simulink model "six_plus_six_AcmsteeringV09_main_2lflm"  (R2014a)
settings: Solver=FixedStepDiscrete  StartTime=0.0  StopTime=10.0  FixedStep=0.0005  RelTol=1e-3
InitFcn:
  | Veh_Par_wxt
undefined symbols (not defined in the file or in its folder): acc_spdctl, ag_thr, B, bra_em, bra_pre_gz2, bra_pre_gz34, bra_pre_yd, brakepre_dem_data, brakeTrq_dem_data, bratrq_max, ecucoder_acal, eff_tran, ESP_switch, G, guzhang_lf, guzhang_lm, guzhang_lr, guzhang_rf, guzhang_rm, guzhang_rr, kd1, kd2, ki1, ki2, kp1, kp2, L, myFIS, premax, Radius, RC_switch, s_opt_yi, s_opt_zhuan, s_opt_zhuan_add, s_opt_zhuan_table, spd_map_mot, spd_spdctl, speed_thr_park, TCS_switch, tras_ratio, trq_map_mot, trqmax_yd, trqmax_zx, trqmaxneg, v_gain, v_table, v_thr_park, zhidong_bianmazhi, zhidong_down, zhidong_up, zhidong_youmen, zhuanxiang_bianmazhi, zhuanxiang_down, zhuanxiang_up, zhuanxiang_youmen
libraries: simulink x980, ec5744lib x59, fuzblock x2
(part 17 of 25)

== system six_plus_six_AcmsteeringV09_main_2lflm/Data_input/BMS5_1/BMS5/BMS5_UpDownRequest_Sub ==
  In1 : Inport
  Out1 : Outport
  wires:
  In1/1 -> Out1/1

== system six_plus_six_AcmsteeringV09_main_2lflm/Data_input/BMS5_2/BMS5/BMS5_15s_InstanceDisPower_Sub ==
  In1 : Inport
  Out1 : Outport
  wires:
  In1/1 -> Out1/1

== system six_plus_six_AcmsteeringV09_main_2lflm/Data_input/BMS5_2/BMS5/BMS5_ContDischargePower_Sub ==
  In1 : Inport
  Out1 : Outport
  wires:
  In1/1 -> Out1/1

== system six_plus_six_AcmsteeringV09_main_2lflm/Data_input/BMS5_2/BMS5/BMS5_FailureLevel_Sub ==
  In1 : Inport
  Out1 : Outport
  wires:
  In1/1 -> Out1/1

== system six_plus_six_AcmsteeringV09_main_2lflm/Data_input/BMS5_2/BMS5/BMS5_FeedbackPower_Sub ==
  In1 : Inport
  Out1 : Outport
  wires:
  In1/1 -> Out1/1

== system six_plus_six_AcmsteeringV09_main_2lflm/Data_input/BMS5_2/BMS5/BMS5_UpDownRequest_Sub ==
  In1 : Inport
  Out1 : Outport
  wires:
  In1/1 -> Out1/1

== system six_plus_six_AcmsteeringV09_main_2lflm/Data_input/MCU0/MCU0/MCU0_ControlMode_Sub ==
  In1 : Inport
  Out1 : Outport
  wires:
  In1/1 -> Out1/1

== system six_plus_six_AcmsteeringV09_main_2lflm/Data_input/MCU0/MCU0/MCU0_EmergShutDown_Sub ==
  In1 : Inport
  Out1 : Outport
  wires:
  In1/1 -> Out1/1

== system six_plus_six_AcmsteeringV09_main_2lflm/Data_input/MCU0/MCU0/MCU0_GearStatus_Sub ==
  In1 : Inport
  Out1 : Outport
  wires:
  In1/1 -> Out1/1

== system six_plus_six_AcmsteeringV09_main_2lflm/Data_input/MCU0/MCU0/MCU0_HighVol_Sub ==
  In1 : Inport
  Out1 : Outport
  wires:
  In1/1 -> Out1/1

== system six_plus_six_AcmsteeringV09_main_2lflm/Data_input/MCU0/MCU0/MCU0_LiftCnt_Sub ==
  In1 : Inport
  Out1 : Outport
  wires:
  In1/1 -> Out1/1

== system six_plus_six_AcmsteeringV09_main_2lflm/Data_input/MCU0/MCU0/MCU0_ShutDowAllow_Sub ==
  In1 : Inport
  Out1 : Outport
  wires:
  In1/1 -> Out1/1

== system six_plus_six_AcmsteeringV09_main_2lflm/Data_input/MCU0/MCU0/MCU0_SpeedFdk_Sub ==
  In1 : Inport
  Out1 : Outport
  wires:
  In1/1 -> Out1/1

== system six_plus_six_AcmsteeringV09_main_2lflm/Data_input/MCU0/MCU0/MCU0_TorqueFdk_Sub ==
  In1 : Inport
  Out1 : Outport
  wires:
  In1/1 -> Out1/1

== system six_plus_six_AcmsteeringV09_main_2lflm/Data_input/MCU0/MCU0/MCU0_TorqueMax_Sub ==
  In1 : Inport
  Out1 : Outport
  wires:
  In1/1 -> Out1/1

== system six_plus_six_AcmsteeringV09_main_2lflm/Data_input/MCU0/MCU0/MCU0_WorkStatus_Sub ==
  In1 : Inport
  Out1 : Outport
  wires:
  In1/1 -> Out1/1

== system six_plus_six_AcmsteeringV09_main_2lflm/Data_input/MCU0_1/MCU0/MCU0_ControlMode_Sub ==
  In1 : Inport
  Out1 : Outport
  wires:
  In1/1 -> Out1/1

== system six_plus_six_AcmsteeringV09_main_2lflm/Data_input/MCU0_1/MCU0/MCU0_EmergShutDown_Sub ==
  In1 : Inport
  Out1 : Outport
  wires:
  In1/1 -> Out1/1

== system six_plus_six_AcmsteeringV09_main_2lflm/Data_input/MCU0_1/MCU0/MCU0_GearStatus_Sub ==
  In1 : Inport
  Out1 : Outport
  wires:
  In1/1 -> Out1/1

== system six_plus_six_AcmsteeringV09_main_2lflm/Data_input/MCU0_1/MCU0/MCU0_HighVol_Sub ==
  In1 : Inport
  Out1 : Outport
  wires:
  In1/1 -> Out1/1

== system six_plus_six_AcmsteeringV09_main_2lflm/Data_input/MCU0_1/MCU0/MCU0_LiftCnt_Sub ==
  In1 : Inport
  Out1 : Outport
  wires:
  In1/1 -> Out1/1

== system six_plus_six_AcmsteeringV09_main_2lflm/Data_input/MCU0_1/MCU0/MCU0_ShutDowAllow_Sub ==
  In1 : Inport
  Out1 : Outport
  wires:
  In1/1 -> Out1/1

== system six_plus_six_AcmsteeringV09_main_2lflm/Data_input/MCU0_1/MCU0/MCU0_SpeedFdk_Sub ==
  In1 : Inport
  Out1 : Outport
  wires:
  In1/1 -> Out1/1

== system six_plus_six_AcmsteeringV09_main_2lflm/Data_input/MCU0_1/MCU0/MCU0_TorqueFdk_Sub ==
  In1 : Inport
  Out1 : Outport
  wires:
  In1/1 -> Out1/1

== system six_plus_six_AcmsteeringV09_main_2lflm/Data_input/MCU0_1/MCU0/MCU0_TorqueMax_Sub ==
  In1 : Inport
  Out1 : Outport
  wires:
  In1/1 -> Out1/1

== system six_plus_six_AcmsteeringV09_main_2lflm/Data_input/MCU0_1/MCU0/MCU0_WorkStatus_Sub ==
  In1 : Inport
  Out1 : Outport
  wires:
  In1/1 -> Out1/1

== system six_plus_six_AcmsteeringV09_main_2lflm/Data_input/MCU0_2/MCU0/MCU0_ControlMode_Sub ==
  In1 : Inport
  Out1 : Outport
  wires:
  In1/1 -> Out1/1

== system six_plus_six_AcmsteeringV09_main_2lflm/Data_input/MCU0_2/MCU0/MCU0_EmergShutDown_Sub ==
  In1 : Inport
  Out1 : Outport
  wires:
  In1/1 -> Out1/1

== system six_plus_six_AcmsteeringV09_main_2lflm/Data_input/MCU0_2/MCU0/MCU0_GearStatus_Sub ==
  In1 : Inport
  Out1 : Outport
  wires:
  In1/1 -> Out1/1

== system six_plus_six_AcmsteeringV09_main_2lflm/Data_input/MCU0_2/MCU0/MCU0_HighVol_Sub ==
  In1 : Inport
  Out1 : Outport
  wires:
  In1/1 -> Out1/1

== system six_plus_six_AcmsteeringV09_main_2lflm/Data_input/MCU0_2/MCU0/MCU0_LiftCnt_Sub ==
  In1 : Inport
  Out1 : Outport
  wires:
  In1/1 -> Out1/1

== system six_plus_six_AcmsteeringV09_main_2lflm/Data_input/MCU0_2/MCU0/MCU0_ShutDowAllow_Sub ==
  In1 : Inport
  Out1 : Outport
  wires:
  In1/1 -> Out1/1

== system six_plus_six_AcmsteeringV09_main_2lflm/Data_input/MCU0_2/MCU0/MCU0_SpeedFdk_Sub ==
  In1 : Inport
  Out1 : Outport
  wires:
  In1/1 -> Out1/1

== system six_plus_six_AcmsteeringV09_main_2lflm/Data_input/MCU0_2/MCU0/MCU0_TorqueFdk_Sub ==
  In1 : Inport
  Out1 : Outport
  wires:
  In1/1 -> Out1/1

== system six_plus_six_AcmsteeringV09_main_2lflm/Data_input/MCU0_2/MCU0/MCU0_TorqueMax_Sub ==
  In1 : Inport
  Out1 : Outport
  wires:
  In1/1 -> Out1/1

== matlab function six_plus_six_AcmsteeringV09_main_2lflm/Data_input/10/Enabled
Subsystem/MATLAB Function ==
  data: data1 input; y output; data2 input; data3 input; data4 input
function y = fcn(data1,data2,data3,data4)
%#codegen
y1=data4*256^3+data3*256^2+data2*256+data1;
y=typecast(uint32(y1),'single');
end
% y = u;

== matlab function six_plus_six_AcmsteeringV09_main_2lflm/InputSignalProcess/MATLAB Function ==
  data: LeftJoystick_UpDown input; acc_dem output single; steer_dem output single; brake_dem output single; LeftJoystick_LeftRight input; RirhtJoystick_UpDown input
function [acc_dem,steer_dem,brake_dem] = fcn(LeftJoystick_UpDown,LeftJoystick_LeftRight,RirhtJoystick_UpDown)
%#codegen
if LeftJoystick_UpDown<=1512
    acc_dem=single((LeftJoystick_UpDown-1512)/(1094-1512)*100);
else
    acc_dem=single((LeftJoystick_UpDown-1512)/(1934-1512)*100*-1);
end

if  LeftJoystick_LeftRight <500 || LeftJoystick_LeftRight >2500
    steer_dem = single(0);
elseif LeftJoystick_LeftRight<=1503
    steer_dem=single((LeftJoystick_LeftRight-1503)/(1084-1503)*100);
else
    steer_dem=single((LeftJoystick_LeftRight-1503)/(1923-1503)*100*-1);
end

brake_dem=single((RirhtJoystick_UpDown-1094)/(1934-1094)*100);

end

== system six_plus_six_AcmsteeringV09_main_2lflm/Data_input/MCU0_2/MCU0/MCU0_WorkStatus_Sub ==
  In1 : Inport
  Out1 : Outport
  wires:
  In1/1 -> Out1/1

== system six_plus_six_AcmsteeringV09_main_2lflm/Data_input/MCU0_3/MCU0/MCU0_ControlMode_Sub ==
  In1 : Inport
  Out1 : Outport
  wires:
  In1/1 -> Out1/1

== system six_plus_six_AcmsteeringV09_main_2lflm/Data_input/MCU0_3/MCU0/MCU0_EmergShutDown_Sub ==
  In1 : Inport
  Out1 : Outport
  wires:
  In1/1 -> Out1/1

== system six_plus_six_AcmsteeringV09_main_2lflm/Data_input/MCU0_3/MCU0/MCU0_GearStatus_Sub ==
  In1 : Inport
  Out1 : Outport
  wires:
  In1/1 -> Out1/1

== system six_plus_six_AcmsteeringV09_main_2lflm/Data_input/MCU0_3/MCU0/MCU0_HighVol_Sub ==
  In1 : Inport
  Out1 : Outport
  wires:
  In1/1 -> Out1/1

== system six_plus_six_AcmsteeringV09_main_2lflm/Data_input/MCU0_3/MCU0/MCU0_LiftCnt_Sub ==
  In1 : Inport
  Out1 : Outport
  wires:
  In1/1 -> Out1/1

== system six_plus_six_AcmsteeringV09_main_2lflm/Data_input/MCU0_3/MCU0/MCU0_ShutDowAllow_Sub ==
  In1 : Inport
  Out1 : Outport
  wires:
  In1/1 -> Out1/1

== system six_plus_six_AcmsteeringV09_main_2lflm/Data_input/MCU0_3/MCU0/MCU0_SpeedFdk_Sub ==
  In1 : Inport
  Out1 : Outport
  wires:
  In1/1 -> Out1/1

== system six_plus_six_AcmsteeringV09_main_2lflm/Data_input/MCU0_3/MCU0/MCU0_TorqueFdk_Sub ==
  In1 : Inport
  Out1 : Outport
  wires:
  In1/1 -> Out1/1

== system six_plus_six_AcmsteeringV09_main_2lflm/Data_input/MCU0_3/MCU0/MCU0_TorqueMax_Sub ==
  In1 : Inport
  Out1 : Outport
  wires:
  In1/1 -> Out1/1

== system six_plus_six_AcmsteeringV09_main_2lflm/Data_input/MCU0_3/MCU0/MCU0_WorkStatus_Sub ==
  In1 : Inport
  Out1 : Outport
  wires:
  In1/1 -> Out1/1

== system six_plus_six_AcmsteeringV09_main_2lflm/Data_input/MCU0_4/MCU0/MCU0_ControlMode_Sub ==
  In1 : Inport
  Out1 : Outport
  wires:
  In1/1 -> Out1/1

== system six_plus_six_AcmsteeringV09_main_2lflm/Data_input/MCU0_4/MCU0/MCU0_EmergShutDown_Sub ==
  In1 : Inport
  Out1 : Outport
  wires:
  In1/1 -> Out1/1

== system six_plus_six_AcmsteeringV09_main_2lflm/Data_input/MCU0_4/MCU0/MCU0_GearStatus_Sub ==
  In1 : Inport
  Out1 : Outport
  wires:
  In1/1 -> Out1/1

== system six_plus_six_AcmsteeringV09_main_2lflm/Data_input/MCU0_4/MCU0/MCU0_HighVol_Sub ==
  In1 : Inport
  Out1 : Outport
  wires:
  In1/1 -> Out1/1

== system six_plus_six_AcmsteeringV09_main_2lflm/Data_input/MCU0_4/MCU0/MCU0_LiftCnt_Sub ==
  In1 : Inport
  Out1 : Outport
  wires:
  In1/1 -> Out1/1

== system six_plus_six_AcmsteeringV09_main_2lflm/Data_input/MCU0_4/MCU0/MCU0_ShutDowAllow_Sub ==
  In1 : Inport
  Out1 : Outport
  wires:
  In1/1 -> Out1/1

== system six_plus_six_AcmsteeringV09_main_2lflm/Data_input/MCU0_4/MCU0/MCU0_SpeedFdk_Sub ==
  In1 : Inport
  Out1 : Outport
  wires:
  In1/1 -> Out1/1

== system six_plus_six_AcmsteeringV09_main_2lflm/Data_input/MCU0_4/MCU0/MCU0_TorqueFdk_Sub ==
  In1 : Inport
  Out1 : Outport
  wires:
  In1/1 -> Out1/1

== system six_plus_six_AcmsteeringV09_main_2lflm/Data_input/MCU0_4/MCU0/MCU0_TorqueMax_Sub ==
  In1 : Inport
  Out1 : Outport
  wires:
  In1/1 -> Out1/1

== system six_plus_six_AcmsteeringV09_main_2lflm/Data_input/MCU0_4/MCU0/MCU0_WorkStatus_Sub ==
  In1 : Inport
  Out1 : Outport
  wires:
  In1/1 -> Out1/1

== system six_plus_six_AcmsteeringV09_main_2lflm/Data_input/MCU0_5/MCU0/MCU0_ControlMode_Sub ==
  In1 : Inport
  Out1 : Outport
  wires:
  In1/1 -> Out1/1

== system six_plus_six_AcmsteeringV09_main_2lflm/Data_input/MCU0_5/MCU0/MCU0_EmergShutDown_Sub ==
  In1 : Inport
  Out1 : Outport
  wires:
  In1/1 -> Out1/1

== system six_plus_six_AcmsteeringV09_main_2lflm/Data_input/MCU0_5/MCU0/MCU0_GearStatus_Sub ==
  In1 : Inport
  Out1 : Outport
  wires:
  In1/1 -> Out1/1

== system six_plus_six_AcmsteeringV09_main_2lflm/Data_input/MCU0_5/MCU0/MCU0_HighVol_Sub ==
  In1 : Inport
  Out1 : Outport
  wires:
  In1/1 -> Out1/1

== system six_plus_six_AcmsteeringV09_main_2lflm/Data_input/MCU0_5/MCU0/MCU0_LiftCnt_Sub ==
  In1 : Inport
  Out1 : Outport
  wires:
  In1/1 -> Out1/1

== system six_plus_six_AcmsteeringV09_main_2lflm/Data_input/MCU0_5/MCU0/MCU0_ShutDowAllow_Sub ==
  In1 : Inport
  Out1 : Outport
  wires:
  In1/1 -> Out1/1

== system six_plus_six_AcmsteeringV09_main_2lflm/Data_input/MCU0_5/MCU0/MCU0_SpeedFdk_Sub ==
  In1 : Inport
  Out1 : Outport
  wires:
  In1/1 -> Out1/1

== system six_plus_six_AcmsteeringV09_main_2lflm/Data_input/MCU0_5/MCU0/MCU0_TorqueFdk_Sub ==
  In1 : Inport
  Out1 : Outport
  wires:
  In1/1 -> Out1/1

== system six_plus_six_AcmsteeringV09_main_2lflm/Data_input/MCU0_5/MCU0/MCU0_TorqueMax_Sub ==
  In1 : Inport
  Out1 : Outport
  wires:
  In1/1 -> Out1/1

== system six_plus_six_AcmsteeringV09_main_2lflm/Data_input/MCU0_5/MCU0/MCU0_WorkStatus_Sub ==
  In1 : Inport
  Out1 : Outport
  wires:
  In1/1 -> Out1/1

== system six_plus_six_AcmsteeringV09_main_2lflm/Data_input/MCU1/MCU1/MCU1_ControlTemp_Sub ==
  In1 : Inport
  Out1 : Outport
  wires:
  In1/1 -> Out1/1

== system six_plus_six_AcmsteeringV09_main_2lflm/Data_input/MCU1/MCU1/MCU1_Idc_Sub ==
  In1 : Inport
  Out1 : Outport
  wires:
  In1/1 -> Out1/1

== system six_plus_six_AcmsteeringV09_main_2lflm/Data_input/MCU1/MCU1/MCU1_MotorTemp_Sub ==
  In1 : Inport
  Out1 : Outport
  wires:
  In1/1 -> Out1/1

== system six_plus_six_AcmsteeringV09_main_2lflm/Data_input/MCU1/MCU1/MCU1_PowerFdk_Sub ==
  In1 : Inport
  Out1 : Outport
  wires:
  In1/1 -> Out1/1

== system six_plus_six_AcmsteeringV09_main_2lflm/Data_input/MCU1/MCU1/MCU1_Udc_Sub ==
  In1 : Inport
  Out1 : Outport
  wires:
  In1/1 -> Out1/1

== system six_plus_six_AcmsteeringV09_main_2lflm/Data_input/MCU1_1/MCU1/MCU1_ControlTemp_Sub ==
  In1 : Inport
  Out1 : Outport
  wires:
  In1/1 -> Out1/1

== system six_plus_six_AcmsteeringV09_main_2lflm/Data_input/MCU1_1/MCU1/MCU1_Idc_Sub ==
  In1 : Inport
  Out1 : Outport
  wires:
  In1/1 -> Out1/1

== system six_plus_six_AcmsteeringV09_main_2lflm/Data_input/MCU1_1/MCU1/MCU1_MotorTemp_Sub ==
  In1 : Inport
  Out1 : Outport
  wires:
  In1/1 -> Out1/1

== system six_plus_six_AcmsteeringV09_main_2lflm/Data_input/MCU1_1/MCU1/MCU1_PowerFdk_Sub ==
  In1 : Inport
  Out1 : Outport
  wires:
  In1/1 -> Out1/1

== system six_plus_six_AcmsteeringV09_main_2lflm/Data_input/MCU1_1/MCU1/MCU1_Udc_Sub ==
  In1 : Inport
  Out1 : Outport
  wires:
  In1/1 -> Out1/1

== system six_plus_six_AcmsteeringV09_main_2lflm/Data_input/MCU1_2/MCU1/MCU1_ControlTemp_Sub ==
  In1 : Inport
  Out1 : Outport
  wires:
  In1/1 -> Out1/1

== system six_plus_six_AcmsteeringV09_main_2lflm/Data_input/MCU1_2/MCU1/MCU1_Idc_Sub ==
  In1 : Inport
  Out1 : Outport
  wires:
  In1/1 -> Out1/1

== system six_plus_six_AcmsteeringV09_main_2lflm/Data_input/MCU1_2/MCU1/MCU1_MotorTemp_Sub ==
  In1 : Inport
  Out1 : Outport
  wires:
  In1/1 -> Out1/1

== system six_plus_six_AcmsteeringV09_main_2lflm/Data_input/MCU1_2/MCU1/MCU1_PowerFdk_Sub ==
  In1 : Inport
  Out1 : Outport
  wires:
  In1/1 -> Out1/1

== system six_plus_six_AcmsteeringV09_main_2lflm/Data_input/MCU1_2/MCU1/MCU1_Udc_Sub ==
  In1 : Inport
  Out1 : Outport
  wires:
  In1/1 -> Out1/1

== system six_plus_six_AcmsteeringV09_main_2lflm/Data_input/MCU1_3/MCU1/MCU1_ControlTemp_Sub ==
  In1 : Inport
  Out1 : Outport
  wires:
  In1/1 -> Out1/1

== system six_plus_six_AcmsteeringV09_main_2lflm/Data_input/MCU1_3/MCU1/MCU1_Idc_Sub ==
  In1 : Inport
  Out1 : Outport
  wires:
  In1/1 -> Out1/1

== system six_plus_six_AcmsteeringV09_main_2lflm/Data_input/MCU1_3/MCU1/MCU1_MotorTemp_Sub ==
  In1 : Inport
  Out1 : Outport
  wires:
  In1/1 -> Out1/1

== system six_plus_six_AcmsteeringV09_main_2lflm/Data_input/MCU1_3/MCU1/MCU1_PowerFdk_Sub ==
  In1 : Inport
  Out1 : Outport
  wires:
  In1/1 -> Out1/1

== system six_plus_six_AcmsteeringV09_main_2lflm/Data_input/MCU1_3/MCU1/MCU1_Udc_Sub ==
  In1 : Inport
  Out1 : Outport
  wires:
  In1/1 -> Out1/1

== system six_plus_six_AcmsteeringV09_main_2lflm/Data_input/MCU1_4/MCU1/MCU1_ControlTemp_Sub ==
  In1 : Inport
  Out1 : Outport
  wires:
  In1/1 -> Out1/1

== system six_plus_six_AcmsteeringV09_main_2lflm/Data_input/MCU1_4/MCU1/MCU1_Idc_Sub ==
  In1 : Inport
  Out1 : Outport
  wires:
  In1/1 -> Out1/1

== system six_plus_six_AcmsteeringV09_main_2lflm/Data_input/MCU1_4/MCU1/MCU1_MotorTemp_Sub ==
  In1 : Inport
  Out1 : Outport
  wires:
  In1/1 -> Out1/1

== system six_plus_six_AcmsteeringV09_main_2lflm/Data_input/MCU1_4/MCU1/MCU1_PowerFdk_Sub ==
  In1 : Inport
  Out1 : Outport
  wires:
  In1/1 -> Out1/1

== system six_plus_six_AcmsteeringV09_main_2lflm/Data_input/MCU1_4/MCU1/MCU1_Udc_Sub ==
  In1 : Inport
  Out1 : Outport
  wires:
  In1/1 -> Out1/1

== system six_plus_six_AcmsteeringV09_main_2lflm/Data_input/MCU1_5/MCU1/MCU1_ControlTemp_Sub ==
  In1 : Inport
  Out1 : Outport
  wires:
  In1/1 -> Out1/1

== system six_plus_six_AcmsteeringV09_main_2lflm/Data_input/MCU1_5/MCU1/MCU1_Idc_Sub ==
  In1 : Inport
  Out1 : Outport
  wires:
  In1/1 -> Out1/1

== system six_plus_six_AcmsteeringV09_main_2lflm/Data_input/MCU1_5/MCU1/MCU1_MotorTemp_Sub ==
  In1 : Inport
  Out1 : Outport
  wires:
  In1/1 -> Out1/1

== system six_plus_six_AcmsteeringV09_main_2lflm/Data_input/MCU1_5/MCU1/MCU1_PowerFdk_Sub ==
  In1 : Inport
  Out1 : Outport
  wires:
  In1/1 -> Out1/1

== system six_plus_six_AcmsteeringV09_main_2lflm/Data_input/MCU1_5/MCU1/MCU1_Udc_Sub ==
  In1 : Inport
  Out1 : Outport
  wires:
  In1/1 -> Out1/1

== system six_plus_six_AcmsteeringV09_main_2lflm/Data_input/MCU2/MCU2/MCU2_ActieDischargingFault_Sub ==
  In1 : Inport
  Out1 : Outport
  wires:
  In1/1 -> Out1/1

== system six_plus_six_AcmsteeringV09_main_2lflm/Data_input/MCU2/MCU2/MCU2_CanCommunicationFault_Sub ==
  In1 : Inport
  Out1 : Outport
  wires:
  In1/1 -> Out1/1

== system six_plus_six_AcmsteeringV09_main_2lflm/Data_input/MCU2/MCU2/MCU2_ControllerOverTemp_Sub ==
  In1 : Inport
  Out1 : Outport
  wires:
  In1/1 -> Out1/1

== system six_plus_six_AcmsteeringV09_main_2lflm/Data_input/MCU2/MCU2/MCU2_ControllerOverload_Sub ==
  In1 : Inport
  Out1 : Outport
  wires:
  In1/1 -> Out1/1

== system six_plus_six_AcmsteeringV09_main_2lflm/Data_input/MCU2/MCU2/MCU2_DownratingFault_Sub ==
  In1 : Inport
  Out1 : Outport
  wires:
  In1/1 -> Out1/1

== system six_plus_six_AcmsteeringV09_main_2lflm/Data_input/MCU2/MCU2/MCU2_FaultLevel_Sub ==
  In1 : Inport
  Out1 : Outport
  wires:
  In1/1 -> Out1/1

== system six_plus_six_AcmsteeringV09_main_2lflm/Data_input/MCU2/MCU2/MCU2_IGBTFault_Sub ==
  In1 : Inport
  Out1 : Outport
  wires:
  In1/1 -> Out1/1

== system six_plus_six_AcmsteeringV09_main_2lflm/Data_input/MCU2/MCU2/MCU2_IdcSensorFault_Sub ==
  In1 : Inport
  Out1 : Outport
  wires:
  In1/1 -> Out1/1

== system six_plus_six_AcmsteeringV09_main_2lflm/Data_input/MCU2/MCU2/MCU2_IuSensorFault_Sub ==
  In1 : Inport
  Out1 : Outport
  wires:
  In1/1 -> Out1/1

== system six_plus_six_AcmsteeringV09_main_2lflm/Data_input/MCU2/MCU2/MCU2_IvSensorFault_Sub ==
  In1 : Inport
  Out1 : Outport
  wires:
  In1/1 -> Out1/1

== system six_plus_six_AcmsteeringV09_main_2lflm/Data_input/MCU2/MCU2/MCU2_MemoryFault_Sub ==
  In1 : Inport
  Out1 : Outport
  wires:
  In1/1 -> Out1/1

== system six_plus_six_AcmsteeringV09_main_2lflm/Data_input/MCU2/MCU2/MCU2_MotorOverLoad_Sub ==
  In1 : Inport
  Out1 : Outport
  wires:
  In1/1 -> Out1/1

== system six_plus_six_AcmsteeringV09_main_2lflm/Data_input/MCU2/MCU2/MCU2_MotorOverSpeed_Sub ==
  In1 : Inport
  Out1 : Outport
  wires:
  In1/1 -> Out1/1

== system six_plus_six_AcmsteeringV09_main_2lflm/Data_input/MCU2/MCU2/MCU2_MotorOverTemp_Sub ==
  In1 : Inport
  Out1 : Outport
  wires:
  In1/1 -> Out1/1

== system six_plus_six_AcmsteeringV09_main_2lflm/Data_input/MCU2/MCU2/MCU2_MotorStallingFault_Sub ==
  In1 : Inport
  Out1 : Outport
  wires:
  In1/1 -> Out1/1

== system six_plus_six_AcmsteeringV09_main_2lflm/Data_input/MCU2/MCU2/MCU2_OverVoltage_Sub ==
  In1 : Inport
  Out1 : Outport
  wires:
  In1/1 -> Out1/1

== system six_plus_six_AcmsteeringV09_main_2lflm/Data_input/MCU2/MCU2/MCU2_RotaryInverterFault_Sub ==
  In1 : Inport
  Out1 : Outport
  wires:
  In1/1 -> Out1/1

== system six_plus_six_AcmsteeringV09_main_2lflm/Data_input/MCU2/MCU2/MCU2_TempSensorFault_Sub ==
  In1 : Inport
  Out1 : Outport
  wires:
  In1/1 -> Out1/1

== system six_plus_six_AcmsteeringV09_main_2lflm/Data_input/MCU2/MCU2/MCU2_UdcDetectionFault_Sub ==
  In1 : Inport
  Out1 : Outport
  wires:
  In1/1 -> Out1/1

== system six_plus_six_AcmsteeringV09_main_2lflm/Data_input/MCU2/MCU2/MCU2_UnderVoltage_Sub ==
  In1 : Inport
  Out1 : Outport
  wires:
  In1/1 -> Out1/1

== system six_plus_six_AcmsteeringV09_main_2lflm/Data_input/MCU2_1/MCU2/MCU2_ActieDischargingFault_Sub ==
  In1 : Inport
  Out1 : Outport
  wires:
  In1/1 -> Out1/1

== system six_plus_six_AcmsteeringV09_main_2lflm/Data_input/MCU2_1/MCU2/MCU2_CanCommunicationFault_Sub ==
  In1 : Inport
  Out1 : Outport
  wires:
  In1/1 -> Out1/1

== system six_plus_six_AcmsteeringV09_main_2lflm/Data_input/MCU2_1/MCU2/MCU2_ControllerOverTemp_Sub ==
  In1 : Inport
  Out1 : Outport
  wires:
  In1/1 -> Out1/1

== system six_plus_six_AcmsteeringV09_main_2lflm/Data_input/MCU2_1/MCU2/MCU2_ControllerOverload_Sub ==
  In1 : Inport
  Out1 : Outport
  wires:
  In1/1 -> Out1/1

== system six_plus_six_AcmsteeringV09_main_2lflm/Data_input/MCU2_1/MCU2/MCU2_DownratingFault_Sub ==
  In1 : Inport
  Out1 : Outport
  wires:
  In1/1 -> Out1/1

== system six_plus_six_AcmsteeringV09_main_2lflm/Data_input/MCU2_1/MCU2/MCU2_FaultLevel_Sub ==
  In1 : Inport
  Out1 : Outport
  wires:
  In1/1 -> Out1/1

== system six_plus_six_AcmsteeringV09_main_2lflm/Data_input/MCU2_1/MCU2/MCU2_IGBTFault_Sub ==
  In1 : Inport
  Out1 : Outport
  wires:
  In1/1 -> Out1/1

== system six_plus_six_AcmsteeringV09_main_2lflm/Data_input/MCU2_1/MCU2/MCU2_IdcSensorFault_Sub ==
  In1 : Inport
  Out1 : Outport
  wires:
  In1/1 -> Out1/1

== system six_plus_six_AcmsteeringV09_main_2lflm/Data_input/MCU2_1/MCU2/MCU2_IuSensorFault_Sub ==
  In1 : Inport
  Out1 : Outport
  wires:
  In1/1 -> Out1/1

== system six_plus_six_AcmsteeringV09_main_2lflm/Data_input/MCU2_1/MCU2/MCU2_IvSensorFault_Sub ==
  In1 : Inport
  Out1 : Outport
  wires:
  In1/1 -> Out1/1

== system six_plus_six_AcmsteeringV09_main_2lflm/Data_input/MCU2_1/MCU2/MCU2_MemoryFault_Sub ==
  In1 : Inport
  Out1 : Outport
  wires:
  In1/1 -> Out1/1

== system six_plus_six_AcmsteeringV09_main_2lflm/Data_input/MCU2_1/MCU2/MCU2_MotorOverLoad_Sub ==
  In1 : Inport
  Out1 : Outport
  wires:
  In1/1 -> Out1/1

== system six_plus_six_AcmsteeringV09_main_2lflm/Data_input/MCU2_1/MCU2/MCU2_MotorOverSpeed_Sub ==
  In1 : Inport
  Out1 : Outport
  wires:
  In1/1 -> Out1/1

== system six_plus_six_AcmsteeringV09_main_2lflm/Data_input/MCU2_1/MCU2/MCU2_MotorOverTemp_Sub ==
  In1 : Inport
  Out1 : Outport
  wires:
  In1/1 -> Out1/1

== system six_plus_six_AcmsteeringV09_main_2lflm/Data_input/MCU2_1/MCU2/MCU2_MotorStallingFault_Sub ==
  In1 : Inport
  Out1 : Outport
  wires:
  In1/1 -> Out1/1

== system six_plus_six_AcmsteeringV09_main_2lflm/Data_input/MCU2_1/MCU2/MCU2_OverVoltage_Sub ==
  In1 : Inport
  Out1 : Outport
  wires:
  In1/1 -> Out1/1

== system six_plus_six_AcmsteeringV09_main_2lflm/Data_input/MCU2_1/MCU2/MCU2_RotaryInverterFault_Sub ==
  In1 : Inport
  Out1 : Outport
  wires:
  In1/1 -> Out1/1

== system six_plus_six_AcmsteeringV09_main_2lflm/Data_input/MCU2_1/MCU2/MCU2_TempSensorFault_Sub ==
  In1 : Inport
  Out1 : Outport
  wires:
  In1/1 -> Out1/1

== system six_plus_six_AcmsteeringV09_main_2lflm/Data_input/MCU2_1/MCU2/MCU2_UdcDetectionFault_Sub ==
  In1 : Inport
  Out1 : Outport
  wires:
  In1/1 -> Out1/1

== system six_plus_six_AcmsteeringV09_main_2lflm/Data_input/MCU2_1/MCU2/MCU2_UnderVoltage_Sub ==
  In1 : Inport
  Out1 : Outport
  wires:
  In1/1 -> Out1/1

== system six_plus_six_AcmsteeringV09_main_2lflm/Data_input/MCU2_2/MCU2/MCU2_ActieDischargingFault_Sub ==
  In1 : Inport
  Out1 : Outport
  wires:
  In1/1 -> Out1/1

== system six_plus_six_AcmsteeringV09_main_2lflm/Data_input/MCU2_2/MCU2/MCU2_CanCommunicationFault_Sub ==
  In1 : Inport
  Out1 : Outport
  wires:
  In1/1 -> Out1/1

== system six_plus_six_AcmsteeringV09_main_2lflm/Data_input/MCU2_2/MCU2/MCU2_ControllerOverTemp_Sub ==
  In1 : Inport
  Out1 : Outport
  wires:
  In1/1 -> Out1/1

== system six_plus_six_AcmsteeringV09_main_2lflm/Data_input/MCU2_2/MCU2/MCU2_ControllerOverload_Sub ==
  In1 : Inport
  Out1 : Outport
  wires:
  In1/1 -> Out1/1

== system six_plus_six_AcmsteeringV09_main_2lflm/Data_input/MCU2_2/MCU2/MCU2_DownratingFault_Sub ==
  In1 : Inport
  Out1 : Outport
  wires:
  In1/1 -> Out1/1

== system six_plus_six_AcmsteeringV09_main_2lflm/Data_input/MCU2_2/MCU2/MCU2_FaultLevel_Sub ==
  In1 : Inport
  Out1 : Outport
  wires:
  In1/1 -> Out1/1

== system six_plus_six_AcmsteeringV09_main_2lflm/Data_input/MCU2_2/MCU2/MCU2_IGBTFault_Sub ==
  In1 : Inport
  Out1 : Outport
  wires:
  In1/1 -> Out1/1

== system six_plus_six_AcmsteeringV09_main_2lflm/Data_input/MCU2_2/MCU2/MCU2_IdcSensorFault_Sub ==
  In1 : Inport
  Out1 : Outport
  wires:
  In1/1 -> Out1/1

== system six_plus_six_AcmsteeringV09_main_2lflm/Data_input/MCU2_2/MCU2/MCU2_IuSensorFault_Sub ==
  In1 : Inport
  Out1 : Outport
  wires:
  In1/1 -> Out1/1

== system six_plus_six_AcmsteeringV09_main_2lflm/Data_input/MCU2_2/MCU2/MCU2_IvSensorFault_Sub ==
  In1 : Inport
  Out1 : Outport
  wires:
  In1/1 -> Out1/1

== system six_plus_six_AcmsteeringV09_main_2lflm/Data_input/MCU2_2/MCU2/MCU2_MemoryFault_Sub ==
  In1 : Inport
  Out1 : Outport
  wires:
  In1/1 -> Out1/1

== system six_plus_six_AcmsteeringV09_main_2lflm/Data_input/MCU2_2/MCU2/MCU2_MotorOverLoad_Sub ==
  In1 : Inport
  Out1 : Outport
  wires:
  In1/1 -> Out1/1

== system six_plus_six_AcmsteeringV09_main_2lflm/Data_input/MCU2_2/MCU2/MCU2_MotorOverSpeed_Sub ==
  In1 : Inport
  Out1 : Outport
  wires:
  In1/1 -> Out1/1

== system six_plus_six_AcmsteeringV09_main_2lflm/Data_input/MCU2_2/MCU2/MCU2_MotorOverTemp_Sub ==
  In1 : Inport
  Out1 : Outport
  wires:
  In1/1 -> Out1/1

== system six_plus_six_AcmsteeringV09_main_2lflm/Data_input/MCU2_2/MCU2/MCU2_MotorStallingFault_Sub ==
  In1 : Inport
  Out1 : Outport
  wires:
  In1/1 -> Out1/1

== system six_plus_six_AcmsteeringV09_main_2lflm/Data_input/MCU2_2/MCU2/MCU2_OverVoltage_Sub ==
  In1 : Inport
  Out1 : Outport
  wires:
  In1/1 -> Out1/1

== system six_plus_six_AcmsteeringV09_main_2lflm/Data_input/MCU2_2/MCU2/MCU2_RotaryInverterFault_Sub ==
  In1 : Inport
  Out1 : Outport
  wires:
  In1/1 -> Out1/1

== system six_plus_six_AcmsteeringV09_main_2lflm/Data_input/MCU2_2/MCU2/MCU2_TempSensorFault_Sub ==
  In1 : Inport
  Out1 : Outport
  wires:
  In1/1 -> Out1/1

== system six_plus_six_AcmsteeringV09_main_2lflm/Data_input/MCU2_2/MCU2/MCU2_UdcDetectionFault_Sub ==
  In1 : Inport
  Out1 : Outport
  wires:
  In1/1 -> Out1/1

== system six_plus_six_AcmsteeringV09_main_2lflm/Data_input/MCU2_2/MCU2/MCU2_UnderVoltage_Sub ==
  In1 : Inport
  Out1 : Outport
  wires:
  In1/1 -> Out1/1

== system six_plus_six_AcmsteeringV09_main_2lflm/Data_input/MCU2_3/MCU2/MCU2_ActieDischargingFault_Sub ==
  In1 : Inport
  Out1 : Outport
  wires:
  In1/1 -> Out1/1

== system six_plus_six_AcmsteeringV09_main_2lflm/Data_input/MCU2_3/MCU2/MCU2_CanCommunicationFault_Sub ==
  In1 : Inport
  Out1 : Outport
  wires:
  In1/1 -> Out1/1

== system six_plus_six_AcmsteeringV09_main_2lflm/Data_input/MCU2_3/MCU2/MCU2_ControllerOverTemp_Sub ==
  In1 : Inport
  Out1 : Outport
  wires:
  In1/1 -> Out1/1

== system six_plus_six_AcmsteeringV09_main_2lflm/Data_input/MCU2_3/MCU2/MCU2_ControllerOverload_Sub ==
  In1 : Inport
  Out1 : Outport
  wires:
  In1/1 -> Out1/1

== system six_plus_six_AcmsteeringV09_main_2lflm/Data_input/MCU2_3/MCU2/MCU2_DownratingFault_Sub ==
  In1 : Inport
  Out1 : Outport
  wires:
  In1/1 -> Out1/1

== system six_plus_six_AcmsteeringV09_main_2lflm/Data_input/MCU2_3/MCU2/MCU2_FaultLevel_Sub ==
  In1 : Inport
  Out1 : Outport
  wires:
  In1/1 -> Out1/1

== system six_plus_six_AcmsteeringV09_main_2lflm/Data_input/MCU2_3/MCU2/MCU2_IGBTFault_Sub ==
  In1 : Inport
  Out1 : Outport
  wires:
  In1/1 -> Out1/1

== system six_plus_six_AcmsteeringV09_main_2lflm/Data_input/MCU2_3/MCU2/MCU2_IdcSensorFault_Sub ==
  In1 : Inport
  Out1 : Outport
  wires:
  In1/1 -> Out1/1

== system six_plus_six_AcmsteeringV09_main_2lflm/Data_input/MCU2_3/MCU2/MCU2_IuSensorFault_Sub ==
  In1 : Inport
  Out1 : Outport
  wires:
  In1/1 -> Out1/1

== system six_plus_six_AcmsteeringV09_main_2lflm/Data_input/MCU2_3/MCU2/MCU2_IvSensorFault_Sub ==
  In1 : Inport
  Out1 : Outport
  wires:
  In1/1 -> Out1/1

== system six_plus_six_AcmsteeringV09_main_2lflm/Data_input/MCU2_3/MCU2/MCU2_MemoryFault_Sub ==
  In1 : Inport
  Out1 : Outport
  wires:
  In1/1 -> Out1/1

== system six_plus_six_AcmsteeringV09_main_2lflm/Data_input/MCU2_3/MCU2/MCU2_MotorOverLoad_Sub ==
  In1 : Inport
  Out1 : Outport
  wires:
  In1/1 -> Out1/1

== system six_plus_six_AcmsteeringV09_main_2lflm/Data_input/MCU2_3/MCU2/MCU2_MotorOverSpeed_Sub ==
  In1 : Inport
  Out1 : Outport
  wires:
  In1/1 -> Out1/1

== system six_plus_six_AcmsteeringV09_main_2lflm/Data_input/MCU2_3/MCU2/MCU2_MotorOverTemp_Sub ==
  In1 : Inport
  Out1 : Outport
  wires:
  In1/1 -> Out1/1

== system six_plus_six_AcmsteeringV09_main_2lflm/Data_input/MCU2_3/MCU2/MCU2_MotorStallingFault_Sub ==
  In1 : Inport
  Out1 : Outport
  wires:
  In1/1 -> Out1/1

== system six_plus_six_AcmsteeringV09_main_2lflm/Data_input/MCU2_3/MCU2/MCU2_OverVoltage_Sub ==
  In1 : Inport
  Out1 : Outport
  wires:
  In1/1 -> Out1/1

== system six_plus_six_AcmsteeringV09_main_2lflm/Data_input/MCU2_3/MCU2/MCU2_RotaryInverterFault_Sub ==
  In1 : Inport
  Out1 : Outport
  wires:
  In1/1 -> Out1/1

== system six_plus_six_AcmsteeringV09_main_2lflm/Data_input/MCU2_3/MCU2/MCU2_TempSensorFault_Sub ==
  In1 : Inport
  Out1 : Outport
  wires:
  In1/1 -> Out1/1

== system six_plus_six_AcmsteeringV09_main_2lflm/Data_input/MCU2_3/MCU2/MCU2_UdcDetectionFault_Sub ==
  In1 : Inport
  Out1 : Outport
  wires:
  In1/1 -> Out1/1

== system six_plus_six_AcmsteeringV09_main_2lflm/Data_input/MCU2_3/MCU2/MCU2_UnderVoltage_Sub ==
  In1 : Inport
  Out1 : Outport
  wires:
  In1/1 -> Out1/1

== system six_plus_six_AcmsteeringV09_main_2lflm/Data_input/MCU2_4/MCU2/MCU2_ActieDischargingFault_Sub ==
  In1 : Inport
  Out1 : Outport
  wires:
  In1/1 -> Out1/1

== system six_plus_six_AcmsteeringV09_main_2lflm/Data_input/MCU2_4/MCU2/MCU2_CanCommunicationFault_Sub ==
  In1 : Inport
  Out1 : Outport
  wires:
  In1/1 -> Out1/1

== system six_plus_six_AcmsteeringV09_main_2lflm/Data_input/MCU2_4/MCU2/MCU2_ControllerOverTemp_Sub ==
  In1 : Inport
  Out1 : Outport
  wires:
  In1/1 -> Out1/1

== system six_plus_six_AcmsteeringV09_main_2lflm/Data_input/MCU2_4/MCU2/MCU2_ControllerOverload_Sub ==
  In1 : Inport
  Out1 : Outport
  wires:
  In1/1 -> Out1/1

== system six_plus_six_AcmsteeringV09_main_2lflm/Data_input/MCU2_4/MCU2/MCU2_DownratingFault_Sub ==
  In1 : Inport
  Out1 : Outport
  wires:
  In1/1 -> Out1/1

== system six_plus_six_AcmsteeringV09_main_2lflm/Data_input/MCU2_4/MCU2/MCU2_FaultLevel_Sub ==
  In1 : Inport
  Out1 : Outport
  wires:
  In1/1 -> Out1/1

== system six_plus_six_AcmsteeringV09_main_2lflm/Data_input/MCU2_4/MCU2/MCU2_IGBTFault_Sub ==
  In1 : Inport
  Out1 : Outport
  wires:
  In1/1 -> Out1/1

== system six_plus_six_AcmsteeringV09_main_2lflm/Data_input/MCU2_4/MCU2/MCU2_IdcSensorFault_Sub ==
  In1 : Inport
  Out1 : Outport
  wires:
  In1/1 -> Out1/1

== system six_plus_six_AcmsteeringV09_main_2lflm/Data_input/MCU2_4/MCU2/MCU2_IuSensorFault_Sub ==
  In1 : Inport
  Out1 : Outport
  wires:
  In1/1 -> Out1/1

== system six_plus_six_AcmsteeringV09_main_2lflm/Data_input/MCU2_4/MCU2/MCU2_IvSensorFault_Sub ==
  In1 : Inport
  Out1 : Outport
  wires:
  In1/1 -> Out1/1

== system six_plus_six_AcmsteeringV09_main_2lflm/Data_input/MCU2_4/MCU2/MCU2_MemoryFault_Sub ==
  In1 : Inport
  Out1 : Outport
  wires:
  In1/1 -> Out1/1

== system six_plus_six_AcmsteeringV09_main_2lflm/Data_input/MCU2_4/MCU2/MCU2_MotorOverLoad_Sub ==
  In1 : Inport
  Out1 : Outport
  wires:
  In1/1 -> Out1/1

== system six_plus_six_AcmsteeringV09_main_2lflm/Data_input/MCU2_4/MCU2/MCU2_MotorOverSpeed_Sub ==
  In1 : Inport
  Out1 : Outport
  wires:
  In1/1 -> Out1/1

== system six_plus_six_AcmsteeringV09_main_2lflm/Data_input/MCU2_4/MCU2/MCU2_MotorOverTemp_Sub ==
  In1 : Inport
  Out1 : Outport
  wires:
  In1/1 -> Out1/1

== system six_plus_six_AcmsteeringV09_main_2lflm/Data_input/MCU2_4/MCU2/MCU2_MotorStallingFault_Sub ==
  In1 : Inport
  Out1 : Outport
  wires:
  In1/1 -> Out1/1

== system six_plus_six_AcmsteeringV09_main_2lflm/Data_input/MCU2_4/MCU2/MCU2_OverVoltage_Sub ==
  In1 : Inport
  Out1 : Outport
  wires:
  In1/1 -> Out1/1

== system six_plus_six_AcmsteeringV09_main_2lflm/Data_input/MCU2_4/MCU2/MCU2_RotaryInverterFault_Sub ==
  In1 : Inport
  Out1 : Outport
  wires:
  In1/1 -> Out1/1

== system six_plus_six_AcmsteeringV09_main_2lflm/Data_input/MCU2_4/MCU2/MCU2_TempSensorFault_Sub ==
  In1 : Inport
  Out1 : Outport
  wires:
  In1/1 -> Out1/1

== system six_plus_six_AcmsteeringV09_main_2lflm/Data_input/MCU2_4/MCU2/MCU2_UdcDetectionFault_Sub ==
  In1 : Inport
  Out1 : Outport
  wires:
  In1/1 -> Out1/1

== system six_plus_six_AcmsteeringV09_main_2lflm/Data_input/MCU2_4/MCU2/MCU2_UnderVoltage_Sub ==
  In1 : Inport
  Out1 : Outport
  wires:
  In1/1 -> Out1/1

== system six_plus_six_AcmsteeringV09_main_2lflm/Data_input/MCU2_5/MCU2/MCU2_ActieDischargingFault_Sub ==
  In1 : Inport
  Out1 : Outport
  wires:
  In1/1 -> Out1/1

== system six_plus_six_AcmsteeringV09_main_2lflm/Data_input/MCU2_5/MCU2/MCU2_CanCommunicationFault_Sub ==
  In1 : Inport
  Out1 : Outport
  wires:
  In1/1 -> Out1/1

== system six_plus_six_AcmsteeringV09_main_2lflm/Data_input/MCU2_5/MCU2/MCU2_ControllerOverTemp_Sub ==
  In1 : Inport
  Out1 : Outport
  wires:
  In1/1 -> Out1/1

== system six_plus_six_AcmsteeringV09_main_2lflm/Data_input/MCU2_5/MCU2/MCU2_ControllerOverload_Sub ==
  In1 : Inport
  Out1 : Outport
  wires:
  In1/1 -> Out1/1

== system six_plus_six_AcmsteeringV09_main_2lflm/Data_input/MCU2_5/MCU2/MCU2_DownratingFault_Sub ==
  In1 : Inport
  Out1 : Outport
  wires:
  In1/1 -> Out1/1

== system six_plus_six_AcmsteeringV09_main_2lflm/Data_input/MCU2_5/MCU2/MCU2_FaultLevel_Sub ==
  In1 : Inport
  Out1 : Outport
  wires:
  In1/1 -> Out1/1

== system six_plus_six_AcmsteeringV09_main_2lflm/Data_input/MCU2_5/MCU2/MCU2_IGBTFault_Sub ==
  In1 : Inport
  Out1 : Outport
  wires:
  In1/1 -> Out1/1

== system six_plus_six_AcmsteeringV09_main_2lflm/Data_input/MCU2_5/MCU2/MCU2_IdcSensorFault_Sub ==
  In1 : Inport
  Out1 : Outport
  wires:
  In1/1 -> Out1/1

== system six_plus_six_AcmsteeringV09_main_2lflm/Data_input/MCU2_5/MCU2/MCU2_IuSensorFault_Sub ==
  In1 : Inport
  Out1 : Outport
  wires:
  In1/1 -> Out1/1

== system six_plus_six_AcmsteeringV09_main_2lflm/Data_input/MCU2_5/MCU2/MCU2_IvSensorFault_Sub ==
  In1 : Inport
  Out1 : Outport
  wires:
  In1/1 -> Out1/1

== system six_plus_six_AcmsteeringV09_main_2lflm/Data_input/MCU2_5/MCU2/MCU2_MemoryFault_Sub ==
  In1 : Inport
  Out1 : Outport
  wires:
  In1/1 -> Out1/1

== system six_plus_six_AcmsteeringV09_main_2lflm/Data_input/MCU2_5/MCU2/MCU2_MotorOverLoad_Sub ==
  In1 : Inport
  Out1 : Outport
  wires:
  In1/1 -> Out1/1

== system six_plus_six_AcmsteeringV09_main_2lflm/Data_input/MCU2_5/MCU2/MCU2_MotorOverSpeed_Sub ==
  In1 : Inport
  Out1 : Outport
  wires:
  In1/1 -> Out1/1

== system six_plus_six_AcmsteeringV09_main_2lflm/Data_input/MCU2_5/MCU2/MCU2_MotorOverTemp_Sub ==
  In1 : Inport
  Out1 : Outport
  wires:
  In1/1 -> Out1/1

== system six_plus_six_AcmsteeringV09_main_2lflm/Data_input/MCU2_5/MCU2/MCU2_MotorStallingFault_Sub ==
  In1 : Inport
  Out1 : Outport
  wires:
  In1/1 -> Out1/1

== system six_plus_six_AcmsteeringV09_main_2lflm/Data_input/MCU2_5/MCU2/MCU2_OverVoltage_Sub ==
  In1 : Inport
  Out1 : Outport
  wires:
  In1/1 -> Out1/1

== system six_plus_six_AcmsteeringV09_main_2lflm/Data_input/MCU2_5/MCU2/MCU2_RotaryInverterFault_Sub ==
  In1 : Inport
  Out1 : Outport
  wires:
  In1/1 -> Out1/1

== system six_plus_six_AcmsteeringV09_main_2lflm/Data_input/MCU2_5/MCU2/MCU2_TempSensorFault_Sub ==
  In1 : Inport
  Out1 : Outport
  wires:
  In1/1 -> Out1/1

== system six_plus_six_AcmsteeringV09_main_2lflm/Data_input/MCU2_5/MCU2/MCU2_UdcDetectionFault_Sub ==
  In1 : Inport
  Out1 : Outport
  wires:
  In1/1 -> Out1/1

== system six_plus_six_AcmsteeringV09_main_2lflm/Data_input/MCU2_5/MCU2/MCU2_UnderVoltage_Sub ==
  In1 : Inport
  Out1 : Outport
  wires:
  In1/1 -> Out1/1

== system six_plus_six_AcmsteeringV09_main_2lflm/Data_input/RemoteControl1/Yaokong2/LIFEspan_Sub ==
  In1 : Inport
  Out1 : Outport
  wires:
  In1/1 -> Out1/1

== system six_plus_six_AcmsteeringV09_main_2lflm/Data_input/RemoteControl1/Yaokong2/SA_Sub ==
  In1 : Inport
  Out1 : Outport
  wires:
  In1/1 -> Out1/1

== system six_plus_six_AcmsteeringV09_main_2lflm/Data_input/RemoteControl1/Yaokong2/SD_Sub ==
  In1 : Inport
  Out1 : Outport
  wires:
  In1/1 -> Out1/1

== system six_plus_six_AcmsteeringV09_main_2lflm/Data_input/RemoteControl1/Yaokong2/SE_Sub ==
  In1 : Inport
  Out1 : Outport
  wires:
  In1/1 -> Out1/1

== system six_plus_six_AcmsteeringV09_main_2lflm/Data_input/RemoteControl1/Yaokong2/SH_Sub ==
  In1 : Inport
  Out1 : Outport
  wires:
  In1/1 -> Out1/1

== system six_plus_six_AcmsteeringV09_main_2lflm/Data_input/RemoteControl2/Yaokong1/Leftstick_leftright_Sub ==
  In1 : Inport
  Out1 : Outport
  wires:
  In1/1 -> Out1/1

== system six_plus_six_AcmsteeringV09_main_2lflm/Data_input/RemoteControl2/Yaokong1/Leftstick_updown_Sub ==
  In1 : Inport
  Out1 : Outport
  wires:
  In1/1 -> Out1/1

== system six_plus_six_AcmsteeringV09_main_2lflm/Data_input/RemoteControl2/Yaokong1/Rightstick_leftright_Sub ==
  In1 : Inport
  Out1 : Outport
  wires:
  In1/1 -> Out1/1

== system six_plus_six_AcmsteeringV09_main_2lflm/Data_input/RemoteControl2/Yaokong1/Rightstick_updown_Sub ==
  In1 : Inport
  Out1 : Outport
  wires:
  In1/1 -> Out1/1

== system six_plus_six_AcmsteeringV09_main_2lflm/MainControl/mode_control/Park/park ==
  Signals : Inport
  1-D Lookup Table1 : Lookup_n-D  NumberOfTableDimensions=1  BreakpointsForDimension1=zhuanxiang_youmen  Table=zhuanxiang_bianmazhi  InternalRulePriority=Speed  RndMeth=Simplest  InputSameDT=on
  1-D Lookup Table2 : Lookup_n-D  NumberOfTableDimensions=1  BreakpointsForDimension1=zhidong_youmen  Table=zhidong_bianmazhi  InternalRulePriority=Speed  RndMeth=Simplest  InputSameDT=on
  Add : Sum
  Bus Selector : BusSelector  OutputSignals=RemoteControl_dem.steer_dem,RemoteControl_dem.brake_dem
  Constant1 : Constant  Value=100000  OutDataTypeStr=single  SampleTime=-1
  Gain : Gain  Gain=0.5
  Gain1 : Gain  Gain=-1
  HeartBeat : MATLAB Function  TreatAsAtomicUnit=on
  HeartBeat1 : MATLAB Function  TreatAsAtomicUnit=on
  HeartBeat2 : MATLAB Function  TreatAsAtomicUnit=on
  HeartBeat3 : MATLAB Function  TreatAsAtomicUnit=on
  HeartBeat4 : MATLAB Function  TreatAsAtomicUnit=on
  HeartBeat5 : MATLAB Function  TreatAsAtomicUnit=on
  Memory{,1..4,6} (6 alike) : Memory  InheritSampleTime=on
  Mux{,1..5} (6 alike) : Mux  Inputs=6
  Saturation : Saturate  UpperLimit=zhuanxiang_up  LowerLimit=zhuanxiang_down
  Saturation1 : Saturate  UpperLimit=zhuanxiang_up  LowerLimit=zhuanxiang_down
  Saturation2 : Saturate  UpperLimit=zhuanxiang_up  LowerLimit=zhuanxiang_down
  Saturation3 : Saturate  UpperLimit=zhidong_up  LowerLimit=zhidong_down
  SpdSet_dem{,1..5} (6 alike) : Constant  Value=0  OutDataTypeStr=single  SampleTime=-1
  TrqSet_dem{,1..5} (6 alike) : Constant  Value=0  OutDataTypeStr=single  SampleTime=-1
  mot_enable{,1..5} (6 alike) : Constant  Value=0  OutDataTypeStr=single  SampleTime=-1
  mot_gear{,1..5} (6 alike) : Constant  Value=0  OutDataTypeStr=single  SampleTime=-1
  mot_mode{,1..5} (6 alike) : Constant  Value=0  OutDataTypeStr=single  SampleTime=-1
  mot_lf : Outport
  mot_lm : Outport  Port=2
  mot_lr : Outport  Port=3
  mot_rf : Outport  Port=4
  mot_rm : Outport  Port=5
  mot_rr : Outport  Port=6
  motec_position_1 : Outport  Port=7
  motec_position_2 : Outport  Port=8
  motec_position_3 : Outport  Port=9
  motec_position_4 : Outport  Port=10
  wires:
  mot_gear/1 -> Mux/3
  mot_mode/1 -> Mux/2
  SpdSet_dem/1 -> Mux/4
  TrqSet_dem/1 -> Mux/5
  Mux/1 -> mot_lf/1
  HeartBeat/1(life) -> Mux/6, Memory/1
  Memory/1 -> HeartBeat/1(life_pre)
  Add/1 -> Saturation3/1
  mot_enable/1 -> Mux/1
  mot_gear1/1 -> Mux2/3
  mot_mode2/1 -> Mux2/2
  SpdSet_dem1/1 -> Mux2/4
  TrqSet_dem1/1 -> Mux2/5
  Mux2/1 -> mot_rf/1
  HeartBeat2/1(life) -> Memory2/1, Mux2/6
  Memory2/1 -> HeartBeat2/1(life_pre)
  mot_enable1/1 -> Mux2/1
  mot_gear2/1 -> Mux4/3
  mot_mode4/1 -> Mux4/2
  SpdSet_dem4/1 -> Mux4/4
  TrqSet_dem4/1 -> Mux4/5
  Mux4/1 -> mot_lm/1
  HeartBeat3/1(life) -> Memory4/1, Mux4/6
  Memory4/1 -> HeartBeat3/1(life_pre)
  mot_enable3/1 -> Mux4/1
  mot_gear3/1 -> Mux5/3
  mot_mode5/1 -> Mux5/2
  SpdSet_dem5/1 -> Mux5/4
  TrqSet_dem5/1 -> Mux5/5
  Mux5/1 -> mot_rm/1
  HeartBeat4/1(life) -> Mux5/6, Memory6/1
  Memory6/1 -> HeartBeat4/1(life_pre)
  mot_enable5/1 -> Mux5/1
  mot_gear4/1 -> Mux1/3
  mot_mode1/1 -> Mux1/2
  SpdSet_dem2/1 -> Mux1/4
  TrqSet_dem2/1 -> Mux1/5
  Mux1/1 -> mot_lr/1
  HeartBeat1/1(life) -> Memory1/1, Mux1/6
  Memory1/1 -> HeartBeat1/1(life_pre)
  mot_enable4/1 -> Mux1/1
  mot_gear5/1 -> Mux3/3
  mot_mode3/1 -> Mux3/2
  SpdSet_dem3/1 -> Mux3/4
  TrqSet_dem3/1 -> Mux3/5
  Mux3/1 -> mot_rr/1
  HeartBeat5/1(life) -> Memory3/1, Mux3/6
  Memory3/1 -> HeartBeat5/1(life_pre)
  mot_enable2/1 -> Mux3/1
  1-D Lookup Table1/1 -> Gain1/1, Gain/1, Saturation/1
  Signals/1 -> Bus Selector/1
  Gain1/1 -> Saturation2/1
  Bus Selector/1 -> 1-D Lookup Table1/1  "<steer_dem>"
  Gain/1 -> Saturation1/1
  Saturation/1 -> motec_position_1/1
  Saturation1/1 -> motec_position_2/1
  Saturation2/1 -> motec_position_3/1
  Saturation3/1 -> motec_position_4/1
  1-D Lookup Table2/1 -> Add/1
  Bus Selector/2 -> 1-D Lookup Table2/1  "<brake_dem>"
  Constant1/1 -> Add/2

== system six_plus_six_AcmsteeringV09_main_2lflm/MainControl/mode_control/backward/backward ==
  Signals : Inport
  Brake : Subsystem  TreatAsAtomicUnit=on
  Bus Selector : BusSelector  OutputSignals=RemoteControl_dem.acc_dem,RemoteControl_dem.brake_dem,RemoteControl_dem.HAC
  Drive : Subsystem  TreatAsAtomicUnit=on
  MATLAB Function : MATLAB Function  TreatAsAtomicUnit=on
  Multiport Switch : MultiPortSwitch  DataPortOrder=Zero-based contiguous  Inputs=2
  Switch Case1 : SwitchCase  CaseConditions={0,1}  ShowDefaultCase=off
  backward_dem : Outport
  wires:
  Signals/1 -> Brake/1(Signals), Drive/1(Signals), Bus Selector/1
  Multiport Switch/1 -> backward_dem/1
  Switch Case1/1 -> Drive/Action
  Switch Case1/2 -> Brake/Action
  Bus Selector/1 -> MATLAB Function/1(acc_dem)  "<acc_dem>"
  MATLAB Function/1(y) -> Multiport Switch/1, Switch Case1/1
  Drive/1(backward_dem) -> Multiport Switch/2
  Brake/1(backward_dem) -> Multiport Switch/3
  Bus Selector/2 -> MATLAB Function/2(brake_dem)  "<brake_dem>"
  Bus Selector/3 -> MATLAB Function/3(HAC)  "<HAC>"
